simulink library "fullCycleController_cl"  (R2020a)
settings: Solver=VariableStepAuto  StartTime=0.0  StopTime=10.0  RelTol=1e-3
undefined symbols (not defined in the file or in its folder): env, FLIGHTCONTROLLER, fltCtrl, initializeBussesFromBlock, vhcl
libraries: filteredPIDController_ul x3, simulink x2, ctrlAllocMatrix_cl x2, dspsigops x1, setpointToOutput_cl x1, pathFollowingController_cl x1
settings Model: Creator=jldanie5  LastModifiedBy=sam3b
settings DataIOCC: ReturnWorkspaceOutputs=off
settings DebuggingCC: ArithmeticOperatorsInVariantConditions=warning
settings SFSimCC: CustomCodeUndefinedFunction=UseInterfaceOnly

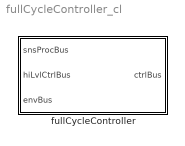
== system fullCycleController_cl ==
  fullCycleController : Subsystem  LoadFcn=initializeBussesFromBlock(gcb)  InitFcn=initializeBussesFromBlock(gcb)  StartFcn=initializeBussesFromBlock(gcb)  VariantControl=strcmpi(FLIGHTCONTROLLER,'takeoffToLanding')  mask{initPosForInitSStar=vhcl.initPosVecGnd.Value, fluidDensity=env.water.density.Value, pathCtrl=fltCtrl, aeroStruct=vhcl.struct('OCT.aeroSurf')}
      mask prompts: initPosForInitSStar "Initial Position"; fluidDensity "Fluid Density"; pathCtrl "Controller"; aeroStruct "Aerodynamic Structure"
      settings: MinAlgLoopOccurrences=on
      mask DialogControl Container3 Prompt: courseFollow Params
      mask DialogControl Container4 Prompt: setpointToOutput Params

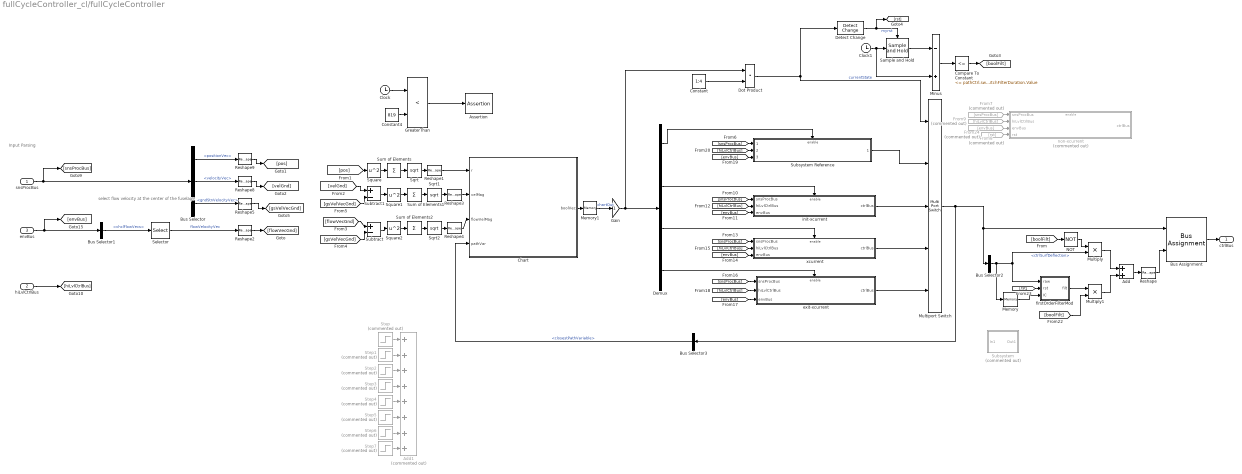
== system fullCycleController_cl/fullCycleController ==
  note: select flow velocity at the center of the fuselage
  note: Input Parsing
  snsProcBus : Inport  OutDataTypeStr=Bus: sensorsProcessingBus
  hiLvlCtrlBus : Inport  Port=2  OutDataTypeStr=Bus: hiLvlCtrlBus
  envBus : Inport  Port=3  OutDataTypeStr=Bus: envBus
  Add : Sum
  Add1 : Sum  Commented=on  Inputs=++++++++
  Assertion : Assertion  Enabled=off  AssertionFailFcn=set_param('OCTModel','SimulationCommand','pause')  StopWhenAssertionFail=off
  Bus Assignment : BusAssignment  AssignedSignals=ctrlSurfDeflection
  Bus Selector : BusSelector  OutputSignals=positionVec,velocityVec,gndStnVelocityVec
  Bus Selector1 : BusSelector  OutputSignals=vhclFlowVecs
  Bus Selector2 : BusSelector  OutputSignals=ctrlSurfDeflection
  Bus Selector3 : BusSelector  OutputSignals=closestPathVariable
  Chart : Stateflow chart  TreatAsAtomicUnit=on  mask{nonCrossSpoolGain=pathCtrl.nonXCurrentSpoolInGain.Value, maxR=pathCtrl.maxTL.Value}
      mask prompts: nonCrossSpoolGain "non-xcurrent spool speed gain"; maxR "max kite position magnitude (r)"
  Clock : Clock
  Clock1 : Clock
  Compare To Constant : simulink/Logic and Bit Operations/Compare To Constant  relop=<=  const=pathCtrl.switchFilterDuration.Value  OutDataTypeStr=boolean
  Constant : Constant  Value=1:4
  Constant4 : Constant  Value=819
  Demux : Demux
  Detect Change : simulink/Logic and Bit Operations/Detect Change  vinit=0  OutDataTypeStr=boolean
  Dot Product : DotProduct  InputSameDT=on  OutDataTypeStr=Inherit: Inherit via internal rule
  From24 : From  Commented=on  GotoTag=rst
  From7 : From  Commented=on  GotoTag=snsProcBus
  From8 : From  Commented=on  GotoTag=envBus
  From9 : From  Commented=on  GotoTag=hiLvlCtrlBus
  Gain : Gain
  GreaterThan : RelationalOperator  Operator=<  OutDataTypeStr=boolean  RndMeth=Simplest
  Memory : Memory  InitialCondition=[0;0;0;0]
  Memory1 : Memory  InitialCondition=[1 0 0 0]
  Minus : Sum  Inputs=-+
  Multiply : Product
  Multiply1 : Product
  Multiport Switch : MultiPortSwitch  Inputs=4  DataPortIndices={1,2,3,4,5,6}  DiagnosticForDefault=Warning
  NOT : Logic  Operator=NOT  AllPortsSameDT=off  OutDataTypeStr=boolean
  Reshape{,1,3..4} (4 alike) : Reshape
  Reshape{2,5,8..9} (4 alike) : Reshape  OutputDimensionality=Column vector (2-D)
  Sample and Hold : dspsigops/Sample and Hold  trig=Rising edge  initCond=0  latchinput=off
  Selector : Selector  NumberOfDimensions=2  InputPortWidth=3  IndexOptions=Select all,Index vector (dialog)  Indices=[1 3],5  OutputSizes=1,1
  Sqrt : Sqrt  SaturateOnIntegerOverflow=on
  Sqrt1 : Sqrt  SaturateOnIntegerOverflow=on
  Sqrt2 : Sqrt  SaturateOnIntegerOverflow=on
  Square : Math  Operator=square  SaturateOnIntegerOverflow=on
  Square1 : Math  Operator=square  SaturateOnIntegerOverflow=on
  Square2 : Math  Operator=square  SaturateOnIntegerOverflow=on
  Step : Step  Commented=on  Time=250  SampleTime=0
  Step1 : Step  Commented=on  Time=260  SampleTime=0
  Step2 : Step  Commented=on  Time=580  SampleTime=0
  Step3 : Step  Commented=on  Time=600  After=-3  SampleTime=0
  Step4 : Step  Commented=on  Time=900  SampleTime=0
  Step5 : Step  Commented=on  Time=910  SampleTime=0
  Step6 : Step  Commented=on  Time=1230  SampleTime=0
  Step7 : Step  Commented=on  Time=1250  After=-3  SampleTime=0
  Subsystem : Subsystem  Commented=on
  Subsystem Reference : Subsystem  ReferencedSubsystem=fullCycleDocked_cl
  Subtract : Sum  Inputs=+-
  Subtract1 : Sum  Inputs=+-
  Sum of Elements : Sum  Inputs=+
  Sum of Elements1 : Sum  Inputs=+
  Sum of Elements2 : Sum  Inputs=+
  exit-xcurrent : Subsystem  TreatAsAtomicUnit=on
  "firstOrderFilterMod " : Subsystem  TreatAsAtomicUnit=on  mask{tau=pathCtrl.switchFilterConstant.Value, ic=0}
      mask prompts: tau "Time Const [s]"; ic "Initial Condition"
      settings: MinAlgLoopOccurrences=on
  init-xcurrent : Subsystem  TreatAsAtomicUnit=on
  non-xcurrent : Subsystem  Commented=on  TreatAsAtomicUnit=on
  xcurrent : Subsystem  TreatAsAtomicUnit=on
  ctrlBus : Outport  OutDataTypeStr=Bus: fltCtrlBus  VectorParamsAs1DForOutWhenUnconnected=off
  wires:
  snsProcBus/1 -> [snsProcBus], Bus Selector/1
  Bus Selector/2 -> Reshape8/1  "<velocityVec>"
  Bus Selector/1 -> Reshape9/1  "<positionVec>"
  Reshape2/1 -> [flowVecGnd]
  Reshape8/1 -> [velGnd]
  Reshape9/1 -> [pos]
  Selector/1 -> Reshape2/1  "flowVelocityVec"
  envBus/1 -> [envBus], Bus Selector1/1
  Bus Selector1/1 -> Selector/1  "<vhclFlowVecs>"
  [pos] -> Square/1
  From8/1 -> non-xcurrent/3(envBus)
  From7/1 -> non-xcurrent/1(snsProcBus)
  From9/1 -> non-xcurrent/2(hiLvlCtrlBus)
  [hiLvlCtrlBus] -> xcurrent/2(hiLvlCtrlBus)
  [snsProcBus] -> xcurrent/1(snsProcBus)
  [envBus] -> xcurrent/3(envBus)
  [hiLvlCtrlBus] -> init-xcurrent/2(hiLvlCtrlBus)
  [envBus] -> init-xcurrent/3(envBus)
  [snsProcBus] -> init-xcurrent/1(snsProcBus)
  [snsProcBus] -> exit-xcurrent/1(snsProcBus)
  [envBus] -> exit-xcurrent/3(envBus)
  [hiLvlCtrlBus] -> exit-xcurrent/2(hiLvlCtrlBus)
  Constant/1 -> Dot Product/2
  Dot Product/1 -> Multiport Switch/1, Detect Change/1  "currentState"
  Chart/1(boolVec) -> Memory1/1
  hiLvlCtrlBus/1 -> [hiLvlCtrlBus]
  Clock/1 -> GreaterThan/1
  Constant4/1 -> GreaterThan/2
  GreaterThan/1 -> Assertion/1
  Clock1/1 -> Minus/2, Sample and Hold/1
  Detect Change/1 -> [rst], Sample and Hold/Trigger  "myrst"
  Sample and Hold/1 -> Minus/1
  Minus/1 -> Compare To Constant/1
  Compare To Constant/1 -> [boolFilt]
  Bus Assignment/1 -> ctrlBus/1
  Multiport Switch/1 -> Bus Selector3/1, Bus Selector2/1, Bus Assignment/1
  Bus Selector2/1 -> Multiply/2, "firstOrderFilterMod "/1(raw), Memory/1  "<ctrlSurfDeflection>"
  [boolFilt] -> NOT/1
  NOT/1 -> Multiply/1
  "firstOrderFilterMod "/1(filt) -> Multiply1/1
  [boolFilt] -> Multiply1/2
  [rst] -> "firstOrderFilterMod "/2(rst)
  Multiply/1 -> Add/1
  Multiply1/1 -> Add/2
  Add/1 -> Reshape/1
  Reshape/1 -> Bus Assignment/2
  Memory/1 -> "firstOrderFilterMod "/3(IC)
  Step/1 -> Add1/1
  Step1/1 -> Add1/2
  Step2/1 -> Add1/3
  Step3/1 -> Add1/4
  From24/1 -> non-xcurrent/4("rst ")
  exit-xcurrent/1(ctrlBus) -> Multiport Switch/5
  xcurrent/1(ctrlBus) -> Multiport Switch/4
  init-xcurrent/1(ctrlBus) -> Multiport Switch/3
  Demux/2 -> init-xcurrent/Enable
  Demux/3 -> xcurrent/Enable
  Demux/4 -> exit-xcurrent/Enable
  Step4/1 -> Add1/5
  Step5/1 -> Add1/6
  Step6/1 -> Add1/7
  Step7/1 -> Add1/8
  Sum of Elements/1 -> Sqrt/1
  Square/1 -> Sum of Elements/1
  Sqrt/1 -> Reshape1/1
  Sum of Elements1/1 -> Sqrt1/1
  Square1/1 -> Sum of Elements1/1
  Sqrt1/1 -> Reshape3/1
  Square2/1 -> Sum of Elements2/1
  Sum of Elements2/1 -> Sqrt2/1
  Sqrt2/1 -> Reshape4/1
  Reshape3/1 -> Chart/2(velMag)
  Reshape4/1 -> Chart/3(flowVelMag)
  Gain/1 -> Dot Product/1, Demux/1
  Memory1/1 -> Gain/1  "chartOut"
  Bus Selector3/1 -> Chart/4(pathVar)  "<closestPathVariable>"
  Bus Selector/3 -> Reshape5/1  "<gndStnVelocityVec>"
  Reshape5/1 -> [gsVelVecGnd]
  [flowVecGnd] -> Subtract/1
  Subtract/1 -> Square2/1
  [gsVelVecGnd] -> Subtract/2
  [gsVelVecGnd] -> Subtract1/2
  Subtract1/1 -> Square1/1
  [velGnd] -> Subtract1/1
  [snsProcBus] -> Subsystem Reference/1
  [hiLvlCtrlBus] -> Subsystem Reference/2
  [envBus] -> Subsystem Reference/3
  Demux/1 -> Subsystem Reference/Enable
  Subsystem Reference/1 -> Multiport Switch/2
  Reshape1/1 -> Chart/1(r)

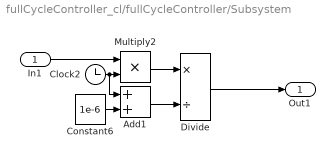
== system fullCycleController_cl/fullCycleController/Subsystem ==
  In1 : Inport
  Add1 : Sum
  Clock2 : Clock
  Constant6 : Constant  Value=1e-6
  Divide : Product  Inputs=*/
  Multiply2 : Product
  Out1 : Outport  VectorParamsAs1DForOutWhenUnconnected=off
  wires:
  In1/1 -> Multiply2/1
  Constant6/1 -> Add1/2
  Clock2/1 -> Add1/1, Multiply2/2
  Divide/1 -> Out1/1
  Multiply2/1 -> Divide/1
  Add1/1 -> Divide/2

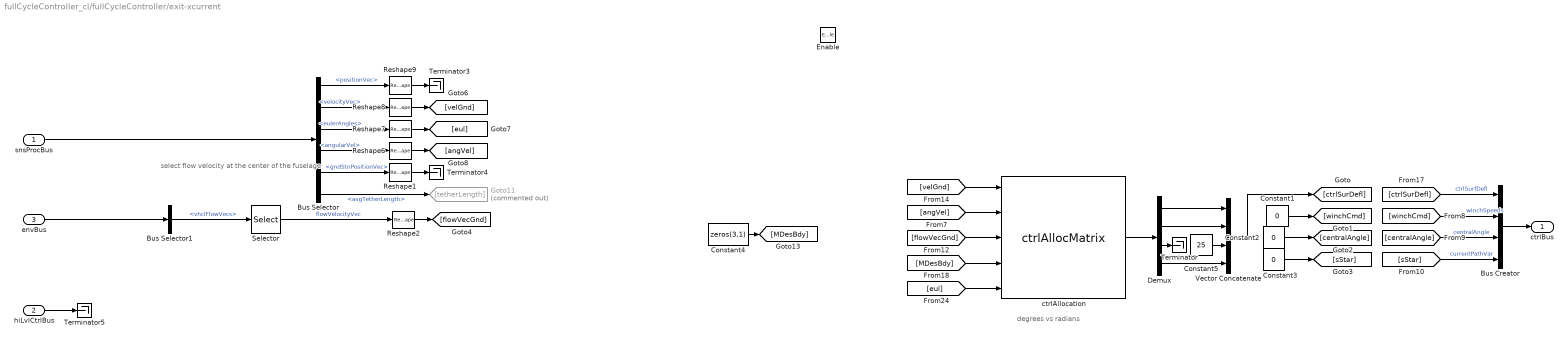
== system fullCycleController_cl/fullCycleController/exit-xcurrent ==
  note: degrees vs radians
  note: select flow velocity at the center of the fuselage
  snsProcBus : Inport  OutDataTypeStr=Bus: sensorsProcessingBus
  hiLvlCtrlBus : Inport  Port=2  OutDataTypeStr=Bus: hiLvlCtrlBus
  envBus : Inport  Port=3  OutDataTypeStr=Bus: envBus
  Enable : EnablePort
  Bus Creator : BusCreator  Inputs=4  OutDataTypeStr=Bus: fltCtrlBus
      settings: InheritFromInputs=off
  Bus Selector : BusSelector  OutputSignals=positionVec,velocityVec,eulerAngles,angularVel,gndStnPositionVec,avgTetherLength
  Bus Selector1 : BusSelector  OutputSignals=vhclFlowVecs
  Constant1 : Constant  Value=0
  Constant2 : Constant  Value=0
  Constant3 : Constant  Value=0
  Constant4 : Constant  Value=zeros(3,1)
  Constant5 : Constant  Value=25
  Demux : Demux
  Goto11 : Goto  Commented=on  GotoTag=tetherLength
  Reshape{1..2,6..9} (6 alike) : Reshape  OutputDimensionality=Column vector (2-D)
  Selector : Selector  NumberOfDimensions=2  InputPortWidth=3  IndexOptions=Select all,Index vector (dialog)  Indices=[1 3],5  OutputSizes=1,1
  Terminator{,3..5} (4 alike) : Terminator
  Vector Concatenate : Concatenate  NumInputs=4
  ctrlAllocation : ctrlAllocMatrix_cl/ctrlAllocMatrix  aeroStruct=aeroStruct  fluidDensity=fluidDensity
  ctrlBus : Outport  OutDataTypeStr=Bus: fltCtrlBus  VectorParamsAs1DForOutWhenUnconnected=off
  wires:
  [sStar] -> Bus Creator/4  "currentPathVar"
  [ctrlSurDefl] -> Bus Creator/1  "ctrlSurfDefl"
  [winchCmd] -> Bus Creator/2  "winchSpeeds"
  Bus Creator/1 -> ctrlBus/1
  [centralAngle] -> Bus Creator/3  "centralAngle"
  Constant1/1 -> [winchCmd]
  Constant2/1 -> [centralAngle]
  Constant3/1 -> [sStar]
  Bus Selector/1 -> Reshape9/1  "<positionVec>"
  Bus Selector/3 -> Reshape7/1  "<eulerAngles>"
  Bus Selector/2 -> Reshape8/1  "<velocityVec>"
  Reshape7/1 -> [eul]
  Bus Selector/4 -> Reshape6/1  "<angularVel>"
  Reshape8/1 -> [velGnd]
  Selector/1 -> Reshape2/1  "flowVelocityVec"
  Reshape9/1 -> Terminator3/1
  Bus Selector/5 -> Reshape1/1  "<gndStnPositionVec>"
  Reshape2/1 -> [flowVecGnd]
  Bus Selector1/1 -> Selector/1  "<vhclFlowVecs>"
  envBus/1 -> Bus Selector1/1
  Reshape1/1 -> Terminator4/1
  snsProcBus/1 -> Bus Selector/1
  Reshape6/1 -> [angVel]
  [flowVecGnd] -> ctrlAllocation/3
  [angVel] -> ctrlAllocation/2
  [eul] -> ctrlAllocation/5
  [MDesBdy] -> ctrlAllocation/4
  [velGnd] -> ctrlAllocation/1
  Bus Selector/6 -> Goto11/1  "<avgTetherLength>"
  ctrlAllocation/1 -> Demux/1
  Vector Concatenate/1 -> [ctrlSurDefl]
  Demux/1 -> Vector Concatenate/1
  Demux/2 -> Vector Concatenate/2
  Demux/4 -> Vector Concatenate/4
  Constant4/1 -> [MDesBdy]
  hiLvlCtrlBus/1 -> Terminator5/1
  Constant5/1 -> Vector Concatenate/3
  Demux/3 -> Terminator/1

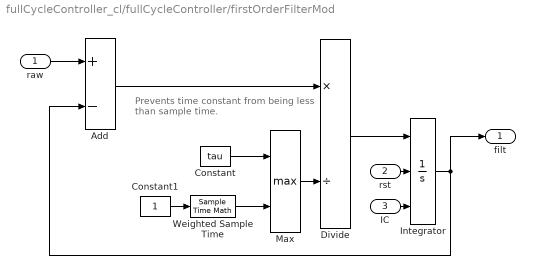
== system fullCycleController_cl/fullCycleController/firstOrderFilterMod  ==
  note: Prevents time constant from
      | being less than sample time.
  raw : Inport
  rst : Inport  Port=2
  IC : Inport  Port=3
  Add : Sum  Inputs=+-
  Constant : Constant  Value=tau
  Constant1 : Constant
  Divide : Product  Inputs=*/
  Integrator : Integrator  ExternalReset=rising  InitialConditionSource=external  InitialCondition=ic
  Max : MinMax  Function=max  Inputs=2
  Weighted Sample Time : SampleTimeMath  TsampMathOp=Ts Only
  filt : Outport  VectorParamsAs1DForOutWhenUnconnected=off
  wires:
  raw/1 -> Add/1
  Add/1 -> Divide/1
  Max/1 -> Divide/2
  Constant/1 -> Max/1
  Constant1/1 -> Weighted Sample Time/1
  Weighted Sample Time/1 -> Max/2
  Divide/1 -> Integrator/1
  Integrator/1 -> Add/2, filt/1
  IC/1 -> Integrator/3
  rst/1 -> Integrator/2

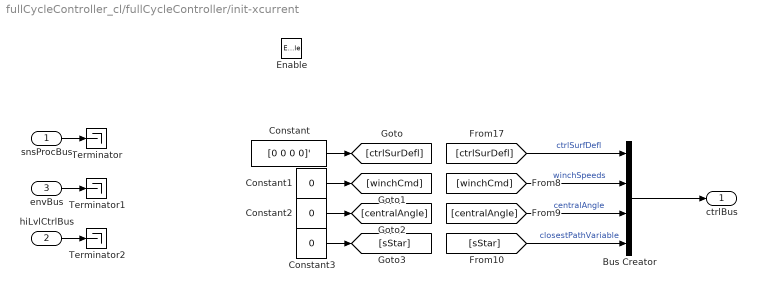
== system fullCycleController_cl/fullCycleController/init-xcurrent ==
  snsProcBus : Inport  OutDataTypeStr=Bus: sensorsProcessingBus
  hiLvlCtrlBus : Inport  Port=2  OutDataTypeStr=Bus: hiLvlCtrlBus
  envBus : Inport  Port=3  OutDataTypeStr=Bus: envBus
  Enable : EnablePort
  Bus Creator : BusCreator  Inputs=4  OutDataTypeStr=Bus: fltCtrlBus
      settings: InheritFromInputs=off
  Constant : Constant  Value=[0 0 0 0]'
  Constant1 : Constant  Value=0
  Constant2 : Constant  Value=0
  Constant3 : Constant  Value=0
  Terminator : Terminator
  Terminator1 : Terminator
  Terminator2 : Terminator
  ctrlBus : Outport  OutDataTypeStr=Bus: fltCtrlBus  VectorParamsAs1DForOutWhenUnconnected=off
  wires:
  [ctrlSurDefl] -> Bus Creator/1  "ctrlSurfDefl"
  [centralAngle] -> Bus Creator/3  "centralAngle"
  [winchCmd] -> Bus Creator/2  "winchSpeeds"
  envBus/1 -> Terminator1/1
  hiLvlCtrlBus/1 -> Terminator2/1
  Constant2/1 -> [centralAngle]
  snsProcBus/1 -> Terminator/1
  [sStar] -> Bus Creator/4  "closestPathVariable"
  Constant1/1 -> [winchCmd]
  Bus Creator/1 -> ctrlBus/1
  Constant3/1 -> [sStar]
  Constant/1 -> [ctrlSurDefl]

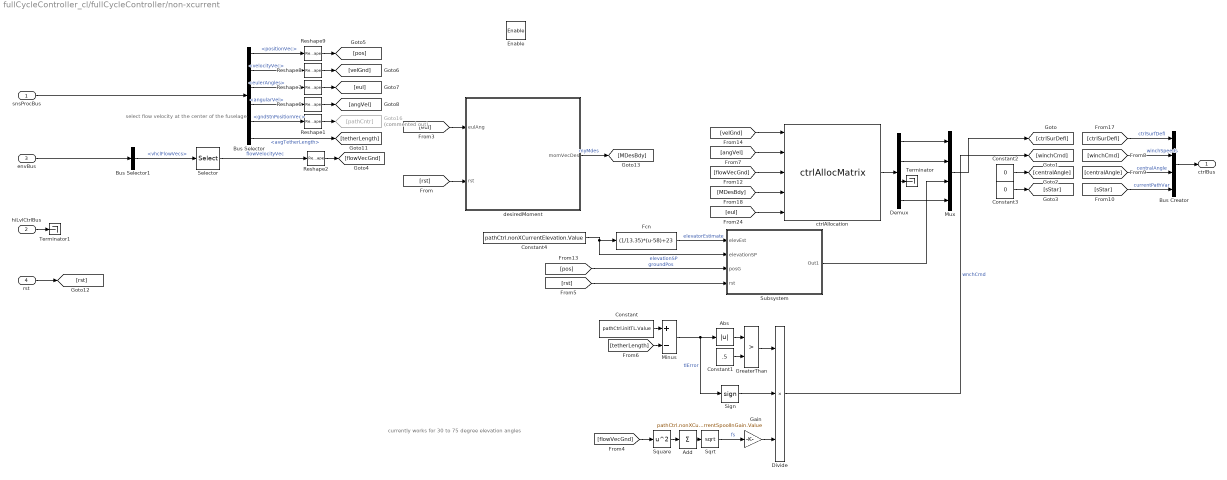
== system fullCycleController_cl/fullCycleController/non-xcurrent ==
  note: select flow velocity at the center of the fuselage
  note: currently works for 30 to 75 degree elevation angles
  snsProcBus : Inport  OutDataTypeStr=Bus: sensorsProcessingBus
  hiLvlCtrlBus : Inport  Port=2  OutDataTypeStr=Bus: hiLvlCtrlBus
  envBus : Inport  Port=3  OutDataTypeStr=Bus: envBus
  "rst " : Inport  Port=4
  Enable : EnablePort
  Abs : Abs
  Add : Sum  Inputs=+
  Bus Creator : BusCreator  Inputs=4  OutDataTypeStr=Bus: fltCtrlBus
      settings: InheritFromInputs=off
  Bus Selector : BusSelector  OutputSignals=positionVec,velocityVec,eulerAngles,angularVel,gndStnPositionVec,avgTetherLength
  Bus Selector1 : BusSelector  OutputSignals=vhclFlowVecs
  Constant : Constant  Value=pathCtrl.initTL.Value
  Constant1 : Constant  Value=.5
  Constant2 : Constant  Value=0
  Constant3 : Constant  Value=0
  Constant4 : Constant  Value=pathCtrl.nonXCurrentElevation.Value
  Demux : Demux
  Divide : Product  Inputs=***
  Fcn : Fcn  Expr=(1/13.35)*(u-58)+23
  Gain : Gain  Gain=pathCtrl.nonXCurrentSpoolInGain.Value
  Goto16 : Goto  Commented=on  GotoTag=pathCntr
  GreaterThan : RelationalOperator  Operator=>  OutDataTypeStr=boolean  RndMeth=Simplest
  Minus : Sum  Inputs=+-
  Mux : Mux
  Reshape{1..2,6..9} (6 alike) : Reshape  OutputDimensionality=Column vector (2-D)
  Selector : Selector  NumberOfDimensions=2  InputPortWidth=3  IndexOptions=Select all,Index vector (dialog)  Indices=[1 3],5  OutputSizes=1,1
  Sign : Signum
  Sqrt : Sqrt  SaturateOnIntegerOverflow=on
  Square : Math  Operator=square  SignedPower=on  SaturateOnIntegerOverflow=on
  Subsystem : Subsystem
  Terminator : Terminator
  Terminator1 : Terminator
  ctrlAllocation : ctrlAllocMatrix_cl/ctrlAllocMatrix  aeroStruct=aeroStruct  fluidDensity=fluidDensity
  desiredMoment : Subsystem
  ctrlBus : Outport  OutDataTypeStr=Bus: fltCtrlBus  VectorParamsAs1DForOutWhenUnconnected=off
  wires:
  [sStar] -> Bus Creator/4  "currentPathVar"
  [ctrlSurDefl] -> Bus Creator/1  "ctrlSurfDefl"
  [winchCmd] -> Bus Creator/2  "winchSpeeds"
  Bus Creator/1 -> ctrlBus/1
  [centralAngle] -> Bus Creator/3  "centralAngle"
  Divide/1 -> [winchCmd]  "wnchCmd"
  Constant2/1 -> [centralAngle]
  Constant3/1 -> [sStar]
  desiredMoment/1(momVecDes) -> [MDesBdy]  "myMdes"
  Bus Selector/1 -> Reshape9/1  "<positionVec>"
  Bus Selector/3 -> Reshape7/1  "<eulerAngles>"
  Bus Selector/2 -> Reshape8/1  "<velocityVec>"
  Reshape7/1 -> [eul]
  Bus Selector/4 -> Reshape6/1  "<angularVel>"
  Reshape8/1 -> [velGnd]
  Selector/1 -> Reshape2/1  "flowVelocityVec"
  Reshape9/1 -> [pos]
  Bus Selector/5 -> Reshape1/1  "<gndStnPositionVec>"
  Reshape2/1 -> [flowVecGnd]
  Bus Selector1/1 -> Selector/1  "<vhclFlowVecs>"
  envBus/1 -> Bus Selector1/1
  Reshape1/1 -> Goto16/1
  snsProcBus/1 -> Bus Selector/1
  Reshape6/1 -> [angVel]
  [eul] -> desiredMoment/1(eulAng)
  [flowVecGnd] -> ctrlAllocation/3
  [angVel] -> ctrlAllocation/2
  [eul] -> ctrlAllocation/5
  [MDesBdy] -> ctrlAllocation/4
  [velGnd] -> ctrlAllocation/1
  [flowVecGnd] -> Square/1
  Add/1 -> Sqrt/1
  Bus Selector/6 -> [tetherLength]  "<avgTetherLength>"
  Constant/1 -> Minus/1
  Minus/1 -> Sign/1, Abs/1  "tlError"
  [tetherLength] -> Minus/2
  Sqrt/1 -> Gain/1  "fs"
  Square/1 -> Add/1
  ctrlAllocation/1 -> Demux/1
  Demux/1 -> Mux/1
  Demux/2 -> Mux/2
  Demux/4 -> Mux/4
  Demux/3 -> Terminator/1
  Constant4/1 -> Fcn/1, Subsystem/2(elevationSP)  "elevationSP"
  Fcn/1 -> Subsystem/1(elevEst)  "elevatorEstimate"
  [pos] -> Subsystem/3(posG)  "groundPos"
  Subsystem/1(Out1) -> Mux/3
  "rst "/1 -> [rst]
  [rst] -> Subsystem/4("rst ")
  hiLvlCtrlBus/1 -> Terminator1/1
  [rst] -> desiredMoment/2(rst)
  Mux/1 -> [ctrlSurDefl]
  Abs/1 -> GreaterThan/1
  Constant1/1 -> GreaterThan/2
  Gain/1 -> Divide/3
  Sign/1 -> Divide/2
  GreaterThan/1 -> Divide/1

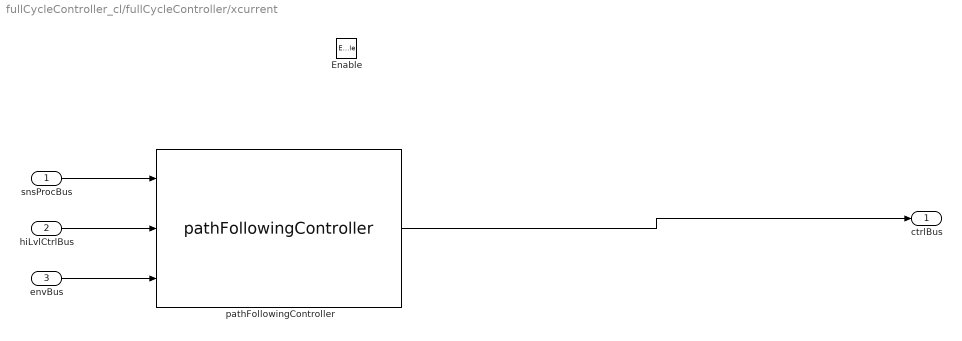
== system fullCycleController_cl/fullCycleController/xcurrent ==
  snsProcBus : Inport  OutDataTypeStr=Bus: sensorsProcessingBus
  hiLvlCtrlBus : Inport  Port=2  OutDataTypeStr=Bus: hiLvlCtrlBus
  envBus : Inport  Port=3  OutDataTypeStr=Bus: envBus
  Enable : EnablePort
  pathFollowingController : pathFollowingController_cl/pathFollowingController  VariantControl=strcmpi(FLIGHTCONTROLLER,'pathFollowingController')  initPosForInitSStar=vhcl.initPosVecGnd.Value  fluidDensity=env.water.density.Value  pathCtrl=fltCtrl  aeroStruct=vhcl.struct('OCT.aeroSurf')
  ctrlBus : Outport  OutDataTypeStr=Bus: fltCtrlBus  VectorParamsAs1DForOutWhenUnconnected=off
  wires:
  snsProcBus/1 -> pathFollowingController/1
  hiLvlCtrlBus/1 -> pathFollowingController/2
  envBus/1 -> pathFollowingController/3
  pathFollowingController/1 -> ctrlBus/1

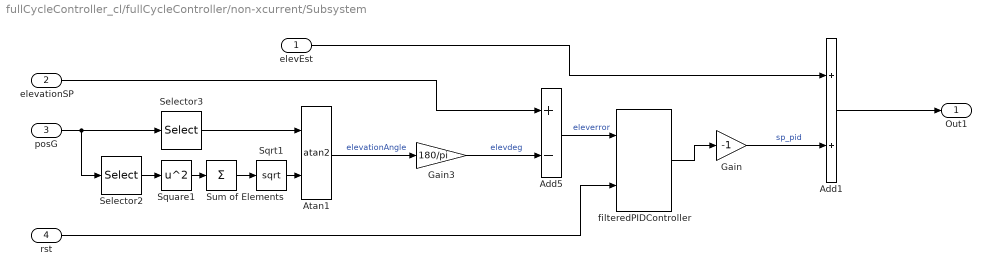
== system fullCycleController_cl/fullCycleController/non-xcurrent/Subsystem ==
  elevEst : Inport
  elevationSP : Inport  Port=2
  posG : Inport  Port=3
  "rst " : Inport  Port=4
  Add1 : Sum
  Add5 : Sum  Inputs=+-
  Atan1 : Trigonometry  Operator=atan2
  Gain : Gain  Gain=-1
  Gain3 : Gain  Gain=180/pi
  Selector2 : Selector  InputPortWidth=3  IndexOptions=Index vector (dialog)  Indices=[1 2]  OutputSizes=1
  Selector3 : Selector  InputPortWidth=3  IndexOptions=Index vector (dialog)  Indices=3  OutputSizes=1
  Sqrt1 : Sqrt  SaturateOnIntegerOverflow=on
  Square1 : Math  Operator=square  SignedPower=on  SaturateOnIntegerOverflow=on
  Sum of Elements : Sum  Inputs=+
  filteredPIDController : filteredPIDController_ul/filteredPIDController  kp=pathCtrl.nonXCurrentElevator.kp.Value  ki=pathCtrl.nonXCurrentElevator.ki.Value  kd=pathCtrl.nonXCurrentElevator.kd.Value  Value=pathCtrl.nonXCurrentElevator.tau.Value  externalReset=rising
  Out1 : Outport  VectorParamsAs1DForOutWhenUnconnected=off
  wires:
  posG/1 -> Selector2/1, Selector3/1
  Square1/1 -> Sum of Elements/1
  Selector2/1 -> Square1/1
  Gain3/1 -> Add5/2  "elevdeg"
  Sqrt1/1 -> Atan1/2
  Selector3/1 -> Atan1/1
  Atan1/1 -> Gain3/1  "elevationAngle"
  Sum of Elements/1 -> Sqrt1/1
  Add5/1 -> filteredPIDController/1  "eleverror"
  Add1/1 -> Out1/1
  elevEst/1 -> Add1/1
  elevationSP/1 -> Add5/1
  "rst "/1 -> filteredPIDController/2
  filteredPIDController/1 -> Gain/1
  Gain/1 -> Add1/2  "sp_pid"

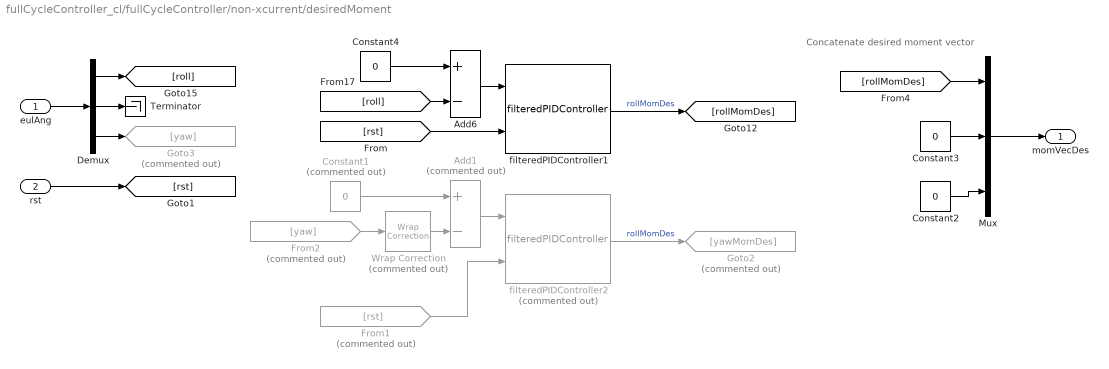
== system fullCycleController_cl/fullCycleController/non-xcurrent/desiredMoment ==
  note: Concatenate desired moment vector
  eulAng : Inport
  rst : Inport  Port=2
  Add1 : Sum  Commented=on  Inputs=+-
  Add6 : Sum  Inputs=+-
  Constant1 : Constant  Commented=on  Value=0
  Constant2 : Constant  Value=0
  Constant3 : Constant  Value=0
  Constant4 : Constant  Value=0
  Demux : Demux  Outputs=3
  From1 : From  Commented=on  GotoTag=rst
  From2 : From  Commented=on  GotoTag=yaw
  Goto2 : Goto  Commented=on  GotoTag=yawMomDes
  Goto3 : Goto  Commented=on  GotoTag=yaw
  Mux : Mux  Inputs=3
  Terminator : Terminator
  Wrap Correction : setpointToOutput_cl/desiredMoment/Wrap Correction  Commented=on  SystemSampleTime=-1  Latency=0  AutoFrameSizeCalculation=off
  filteredPIDController1 : filteredPIDController_ul/filteredPIDController  kp=pathCtrl.rollMoment.kp.Value  ki=0  kd=pathCtrl.rollMoment.kd.Value  Value=pathCtrl.rollMoment.tau.Value  externalReset=rising
  filteredPIDController2 : filteredPIDController_ul/filteredPIDController  Commented=on  kp=pathCtrl.yawMoment.kp.Value  ki=0  kd=pathCtrl.yawMoment.kd.Value  Value=pathCtrl.yawMoment.tau.Value  externalReset=rising
  momVecDes : Outport  VectorParamsAs1DForOutWhenUnconnected=off
  wires:
  Constant2/1 -> Mux/3
  [rollMomDes] -> Mux/1
  Constant3/1 -> Mux/2
  Mux/1 -> momVecDes/1
  Demux/1 -> [roll]
  eulAng/1 -> Demux/1
  filteredPIDController1/1 -> [rollMomDes]  "rollMomDes"
  Add6/1 -> filteredPIDController1/1
  [roll] -> Add6/2
  Constant4/1 -> Add6/1
  Demux/2 -> Terminator/1
  Demux/3 -> Goto3/1
  rst/1 -> [rst]
  [rst] -> filteredPIDController1/2
  From1/1 -> filteredPIDController2/2
  Add1/1 -> filteredPIDController2/1
  filteredPIDController2/1 -> Goto2/1  "rollMomDes"
  Constant1/1 -> Add1/1
  From2/1 -> Wrap Correction/1
  Wrap Correction/1 -> Add1/2

== stateflow chart fullCycleController_cl/fullCycleController/Chart ==
  state Docked
    boolVec=[1 0 0 0];
  (default) -> Docked
  data: boolVec output; r input; velMag input; flowVelMag input; nonCrossSpoolGain parameter; maxR parameter; pathVar input
